simulink model "pendubot_math_plant"  (R2024b)
settings: Solver=ode4  StartTime=0.0  StopTime=2  FixedStep=0.001  RelTol=1e-3
values from neighbouring files (symbols this model uses):
  D = [a + 2*b*cos(q2), d + b*cos(q2) ... (first row only)    [pendubot_dyn.m]
libraries: sharedTrackingLibrary x1
settings Model: Creator=19075  LastModifiedBy=19075

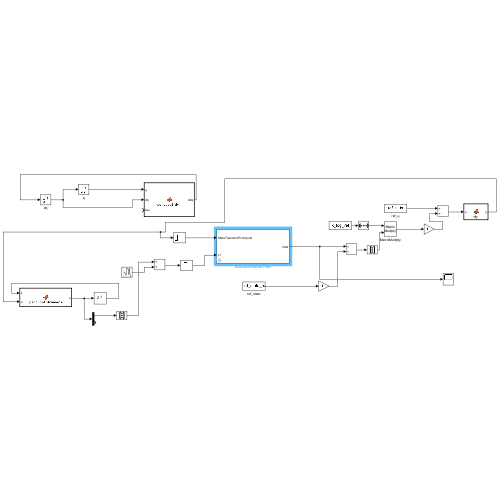
[thumbnail: Simulink's stored preview of the top-level diagram]
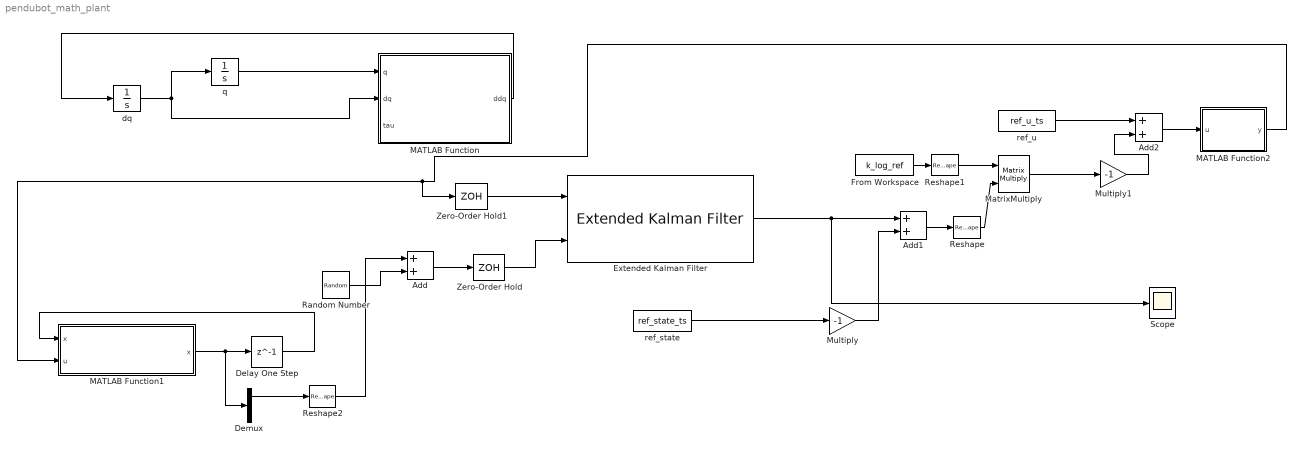
== system pendubot_math_plant ==
  Add : Sum
  Add1 : Sum
  Add2 : Sum
  Delay One Step : Delay  DelayLength=1  InitialCondition=[0;0;0;0]
  Demux : Demux  Outputs=[2 2]
  Extended Kalman Filter : sharedTrackingLibrary/Extended Kalman Filter  StateTransitionFcn=pendubot_f  HasStateTransitionJacobianFcn=off  HasAdditiveProcessNoise=Additive  ProcessNoise=0  HasTimeVaryingProcessNoise=off  HasStateTransitionFcnExtraArgument=1  InitialState=[0;0;0;0]  InitialStateCovariance=1e-6  MeasurementFcn1=pendubot_h  HasMeasurementJacobianFcn1=off  HasMeasurementEnablePort1=off  HasAdditiveMeasurementNoise1=Additive  MeasurementNoise1=diag([0.1 0.1])  HasTimeVaryingMeasurementNoise1=off  HasMeasurementFcnExtraArgument1=0  HasMeasurementWrapping1=off  MeasurementFcn2=myMeasurementFcn  HasMeasurementJacobianFcn2=off  HasMeasurementEnablePort2=off  HasAdditiveMeasurementNoise2=Additive  MeasurementNoise2=1  HasTimeVaryingMeasurementNoise2=off  HasMeasurementFcnExtraArgument2=0  HasMeasurementWrapping2=off  MeasurementFcn3=myMeasurementFcn  HasMeasurementJacobianFcn3=off  HasMeasurementEnablePort3=off  HasAdditiveMeasurementNoise3=Additive  MeasurementNoise3=1  HasTimeVaryingMeasurementNoise3=off  HasMeasurementFcnExtraArgument3=0  HasMeasurementWrapping3=off  MeasurementFcn4=myMeasurementFcn  HasMeasurementJacobianFcn4=off  HasMeasurementEnablePort4=off  HasAdditiveMeasurementNoise4=Additive  MeasurementNoise4=1  HasTimeVaryingMeasurementNoise4=off  HasMeasurementFcnExtraArgument4=0  HasMeasurementWrapping4=off  MeasurementFcn5=myMeasurementFcn  HasMeasurementJacobianFcn5=off  HasMeasurementEnablePort5=off  HasAdditiveMeasurementNoise5=Additive  MeasurementNoise5=1  HasTimeVaryingMeasurementNoise5=off  HasMeasurementFcnExtraArgument5=0  HasMeasurementWrapping5=off  EnableMultirate=off  StateTransitionFcnSampleTime=1  MeasurementFcn1SampleTime=1  MeasurementFcn2SampleTime=1  MeasurementFcn3SampleTime=1  MeasurementFcn4SampleTime=1  MeasurementFcn5SampleTime=1  UseCurrentEstimator=on  OutputStateCovariance=off  DataType=double  SampleTime=0.01  NumberOfMeasurements=1
  From Workspace : FromWorkspace  VariableName=k_log_ref  OutputAfterFinalValue=Holding final value
  MATLAB Function : MATLAB Function  TreatAsAtomicUnit=on
  MATLAB Function1 : MATLAB Function  TreatAsAtomicUnit=on  SystemSampleTime=0.01
  MATLAB Function2 : MATLAB Function  TreatAsAtomicUnit=on
  MatrixMultiply : Product  Multiplication=Matrix(*)
  Multiply : Gain  Gain=-1
  Multiply1 : Gain  Gain=-1
  Random Number : RandomNumber  Variance=0.1  SampleTime=0.01  VectorParams1D=off
  Reshape : Reshape  OutputDimensionality=Column vector (2-D)
  Reshape1 : Reshape  OutputDimensionality=Row vector (2-D)
  Reshape2 : Reshape  OutputDimensionality=Column vector (2-D)
  Scope : Scope
  Zero-Order Hold : ZeroOrderHold  SampleTime=0.01
  Zero-Order Hold1 : ZeroOrderHold  SampleTime=0.01
  dq : Integrator  InitialCondition=[0;0]  LimitOutput=on  ContinuousStateAttributes='velocity'
  q : Integrator  InitialCondition=[0;0]  LimitOutput=on  ContinuousStateAttributes='position'
  ref_state : FromWorkspace  VariableName=ref_state_ts  OutputAfterFinalValue=Holding final value
  ref_u : FromWorkspace  VariableName=ref_u_ts  OutputAfterFinalValue=Setting to zero
  wires:
  dq/1 -> q/1, MATLAB Function/2(dq)
  MATLAB Function/1(ddq) -> dq/1
  Random Number/1 -> Add/2
  Extended Kalman Filter/1 -> Scope/1, Add1/1
  MatrixMultiply/1 -> Multiply1/1
  Multiply1/1 -> Add2/2
  Add1/1 -> Reshape/1
  Reshape/1 -> MatrixMultiply/2
  From Workspace/1 -> Reshape1/1
  Reshape1/1 -> MatrixMultiply/1
  ref_state/1 -> Multiply/1
  Multiply/1 -> Add1/2
  Add2/1 -> MATLAB Function2/1(u)
  MATLAB Function2/1(y) -> Zero-Order Hold1/1, MATLAB Function1/2(u)
  q/1 -> MATLAB Function/1(q)
  MATLAB Function1/1(x) -> Demux/1, Delay One Step/1
  Delay One Step/1 -> MATLAB Function1/1("x ")
  ref_u/1 -> Add2/1
  Demux/1 -> Reshape2/1
  Reshape2/1 -> Add/1
  Add/1 -> Zero-Order Hold/1
  Zero-Order Hold/1 -> Extended Kalman Filter/2
  Zero-Order Hold1/1 -> Extended Kalman Filter/1

== matlab function pendubot_math_plant/MATLAB Function ==
  data: q input; ddq output; dq input; tau input
function ddq = pendubot_dyn(q, dq, tau)
% PENDUBOT_DYN  Pendubot dynamics: D(q) ddq + C(q,dq) dq + G(q) = [tau; 0]
% q  : [q1; q2]
% dq : [dq1; dq2]
% tau: scalar torque at joint 1
% ddq: [ddq1; ddq2]

% ---------- Parameters ----------
dyn.m1 = 1;       % kg
dyn.m2 = 1;       % kg
dyn.l1 = 0.5;     % m
dyn.l2 = 0.5;     % m
dyn.g  = 9.81;    % m/s^2

m1 = dyn.m1; m2 = dyn.m2;
l1 = dyn.l1; l2 = dyn.l2;
g  = dyn.g;

% assume uniform rods
lc1 = l1/2; lc2 = l2/2;
I1  = (1/12)*m1*l1^2;
I2  = (1/12)*m2*l2^2;

% shorthand
q1  = q(1)-pi/2;  q2  = q(2)-q(1);
dq1 = dq(1); dq2 = dq(2);

% ---------- Inertia matrix D(q) ----------
a = I1 + I2 + m1*lc1^2 + m2*(l1^2 + lc2^2);
b = m2*l1*lc2;
d = I2 + m2*lc2^2;

D = [a + 2*b*cos(q2), d + b*cos(q2);
     d + b*cos(q2),   d];

% ---------- Coriolis / centrifugal term C(q,dq)*dq (as a vector) ----------
Cvec = [-b*sin(q2)*(2*dq1 + dq2)*dq2;
         b*sin(q2)*dq1^2];

% ---------- Gravity term G(q) ----------
e = m1*lc1 + m2*l1;
f = m2*lc2;

Gvec = g * [ e*cos(q1) + f*cos(q1+q2);
             f*cos(q1+q2) ];

% ---------- Solve for ddq ----------
Tau = [tau; 0];          % only joint 1 is actuated
ddq = D \ (Tau - Cvec - Gvec);
end

== matlab function pendubot_math_plant/MATLAB Function2 ==
  data: u input; y output
function y = clip(u)

y = max(min(u, 10), -10);
% y=u;
end

== matlab function pendubot_math_plant/MATLAB Function1 ==
  data: x input; u input; x output
function x = pendubot_dynamics(x,u)
% x = [q1; q2; dq1; dq2]
% u = scalar torque
dyn.m1 = 1;  % elbow mass
dyn.m2 = 1; % wrist mass
dyn.g = 9.81;  % gravity
dyn.l1 = 0.5;   % length of first link
dyn.l2 = 0.5;   % length of second link
dt = 0.01;
k1 = pendubotDynamics(x, u, dyn);
k2 = pendubotDynamics(x + 0.5*dt*k1, u, dyn);
k3 = pendubotDynamics(x + 0.5*dt*k2, u, dyn);
k4 = pendubotDynamics(x + dt*k3, u, dyn);
x = x + dt*(k1+2*k2+2*k3+k4)/6;
x(1) = wrapToPi(x(1));
x(2) = wrapToPi(x(2));
end
